simulink model "mainSimulink_localPi"  (R2021a)
settings: Solver=VariableStepAuto  StartTime=0.0  StopTime=inf  FixedStep=sensorSamplingTime  RelTol=1e-3
model workspace (MATLAB code in the model file):
  | %% Simulink settings
  | controllerFile = 'directFFcontroller';
  | set_param('mainSimulink_localPi/Subsystem Reference', 'ReferencedSubsystem', controllerFile);
  | %% Display settings
  | scopeTimeSpan = 30;
  | 
  | %% Robot settings (must match Python)
  | sensorFreq = 125;
  | actuatorFreq = 125;
  | TCPport = 12345;
  | dataSize = 4;
  | sensorSamplingTime = 1/sensorFreq;
  | actuatorTime = 1/actuatorFreq;
undefined symbols (not defined in the file): f
libraries: simulink x2, instrumentlib x2
settings Model: Creator=chukh  LastModifiedBy=brandon

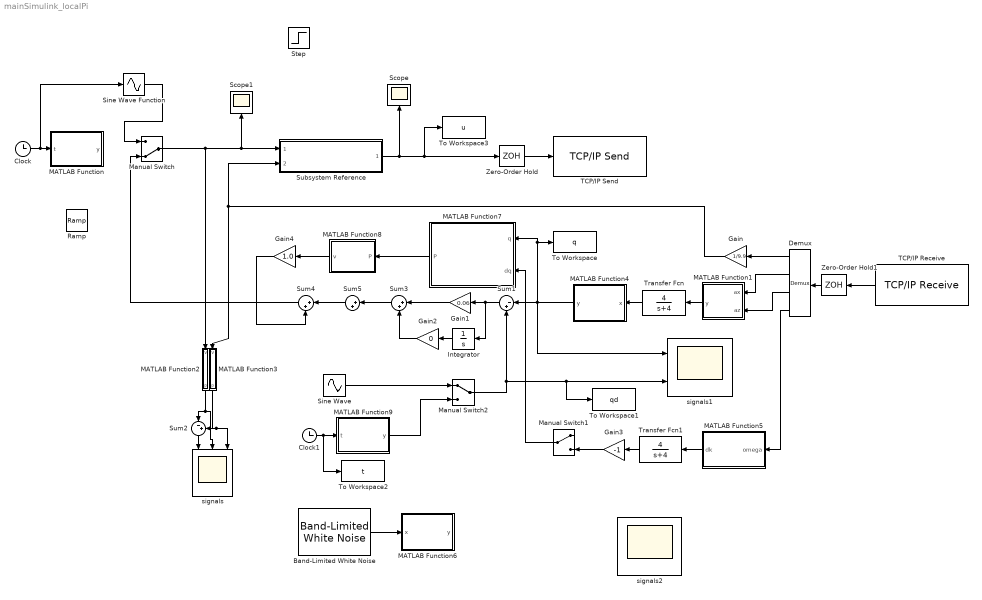
== system mainSimulink_localPi ==
  Band-Limited White Noise : simulink/Sources/Band-Limited White Noise  Cov=[0.1]  Ts=3  seed=[23341]
  Clock : Clock
  Clock1 : Clock
  Demux : Demux
  Gain : Gain  Gain=1/9.9
  Gain1 : Gain  Gain=0.06
  Gain2 : Gain  Gain=0
  Gain3 : Gain  Gain=-1
  Gain4 : Gain  Gain=1.0
  Integrator : Integrator
  MATLAB Function : MATLAB Function  TreatAsAtomicUnit=on
  MATLAB Function1 : MATLAB Function  TreatAsAtomicUnit=on
  MATLAB Function2 : MATLAB Function  TreatAsAtomicUnit=on
  MATLAB Function3 : MATLAB Function  TreatAsAtomicUnit=on
  MATLAB Function4 : MATLAB Function  TreatAsAtomicUnit=on
  MATLAB Function5 : MATLAB Function  TreatAsAtomicUnit=on
  MATLAB Function6 : MATLAB Function  TreatAsAtomicUnit=on
  MATLAB Function7 : MATLAB Function  TreatAsAtomicUnit=on
  MATLAB Function8 : MATLAB Function  TreatAsAtomicUnit=on
  MATLAB Function9 : MATLAB Function  TreatAsAtomicUnit=on
  Manual Switch : ManualSwitch  CurrentSetting=0
  Manual Switch1 : ManualSwitch
  Manual Switch2 : ManualSwitch
  Ramp : simulink/Sources/Ramp  slope=0.06  start=3  InitialOutput=0.6
  Scope : Scope
  Scope1 : Scope
  Sine Wave : Sin  Amplitude=8  Bias=8  Frequency=2  SampleTime=0
  Sine Wave Function : Sin  TimeSource=Use external signal  Amplitude=.4  Bias=0.5  Frequency=2  SampleTime=0
  Step : Step  Time=4  Before=0.6  After=0.85  SampleTime=0
  Subsystem Reference : Subsystem  ReferencedSubsystem=directFFcontroller
  Sum1 : Sum  Inputs=|-+
  Sum2 : Sum  Inputs=|-+
  Sum3 : Sum  Inputs=|++
  Sum4 : Sum  Inputs=|++
  Sum5 : Sum  Inputs=|++
  TCP/IP Receive : instrumentlib/TCP//IP Receive  Host=192.168.4.1  Port=12345  DataSize=dataSize  EnableBlockingMode=on  Timeout=0.5  SampleTime=sensorSamplingTime  DataType=double  ByteOrder=LittleEndian  ASCIIFormatting=%f,  Terminator=LF
  TCP/IP Send : instrumentlib/TCP//IP Send  Host=192.168.4.1  Port=12345  EnableBlockingMode=on  Timeout=0.5  ByteOrder=LittleEndian  TransferDelay=on
  To Workspace : ToWorkspace  VariableName=q  SaveFormat=Timeseries  SampleTime=-1
  To Workspace1 : ToWorkspace  VariableName=qd  SaveFormat=Timeseries  SampleTime=-1
  To Workspace2 : ToWorkspace  VariableName=t  SaveFormat=Timeseries  SampleTime=-1
  To Workspace3 : ToWorkspace  VariableName=u  SaveFormat=Timeseries  SampleTime=-1
  Transfer Fcn : TransferFcn  Numerator=[4]  Denominator=[1 4]
  Transfer Fcn1 : TransferFcn  Numerator=[4]  Denominator=[1 4]
  Zero-Order Hold : ZeroOrderHold  SampleTime=actuatorTime
  Zero-Order Hold1 : ZeroOrderHold  SampleTime=actuatorTime
  signals : Scope  NumInputPorts=3
  signals1 : Scope  NumInputPorts=2
  signals2 : Scope  NumInputPorts=2
  wires:
  Subsystem Reference/1 -> To Workspace3/1, Zero-Order Hold/1, Scope/1
  TCP/IP Receive/1 -> Zero-Order Hold1/1
  Zero-Order Hold/1 -> TCP/IP Send/1
  MATLAB Function2/1(p) -> Sum2/1, signals/2
  Gain/1 -> MATLAB Function3/1(V), Subsystem Reference/2
  MATLAB Function3/1(p) -> Sum2/2, signals/3
  Sum2/1 -> signals/1
  Clock/1 -> Sine Wave Function/1, MATLAB Function/1(t)
  Manual Switch/1 -> Scope1/1, Subsystem Reference/1, MATLAB Function2/1(V)
  Sine Wave Function/1 -> Manual Switch/1
  Demux/1 -> Gain/1
  Zero-Order Hold1/1 -> Demux/1
  Demux/2 -> MATLAB Function1/1(ax)
  MATLAB Function1/1(y) -> Transfer Fcn/1
  Transfer Fcn/1 -> MATLAB Function4/1(x)
  MATLAB Function4/1(y) -> MATLAB Function7/1(q), To Workspace/1, Sum1/1, signals1/1
  Sum1/1 -> Integrator/1, Gain1/1
  Integrator/1 -> Gain2/1
  Gain1/1 -> Sum3/1
  Gain2/1 -> Sum3/2
  Demux/3 -> MATLAB Function1/2(az)
  Sum4/1 -> Manual Switch/2
  Demux/4 -> MATLAB Function5/1(omega)
  MATLAB Function5/1(dk) -> Transfer Fcn1/1
  Band-Limited White Noise/1 -> MATLAB Function6/1(x)
  MATLAB Function7/1(P) -> MATLAB Function8/1(P)
  MATLAB Function8/1(v) -> Gain4/1
  Gain4/1 -> Sum4/2
  Sum3/1 -> Sum5/1
  Sum5/1 -> Sum4/1
  Manual Switch1/1 -> MATLAB Function7/2(dq)
  Gain3/1 -> Manual Switch1/2
  Transfer Fcn1/1 -> Gain3/1
  Sine Wave/1 -> Manual Switch2/1
  MATLAB Function9/1(y) -> Manual Switch2/2
  Manual Switch2/1 -> Sum1/2, To Workspace1/1, signals1/2
  Clock1/1 -> To Workspace2/1, MATLAB Function9/1(t)

== matlab function mainSimulink_localPi/MATLAB Function2 ==
  data: V input; p output
function p = V2kPa(V)
p = (V-0.5)*200;

== matlab function mainSimulink_localPi/MATLAB Function3 ==
  data: V input; p output
function p = V2kPa(V)
p = (V-0.5)*200;

== matlab function mainSimulink_localPi/MATLAB Function1 ==
  data: ax input; y output; az input
function y = fcn(ax,az)

y = -atan2(-az,-ax);

== matlab function mainSimulink_localPi/MATLAB Function4 ==
  data: x input; y output
function y = rad2kappa(x)
y = x/0.0875;
end

== matlab function mainSimulink_localPi/MATLAB Function5 ==
  data: omega input; dk output
function dk = fcn(omega)

dk = omega/0.085;

== matlab function mainSimulink_localPi/MATLAB Function6 ==
  data: x input; y output
function y = rad2kappa(x)
y = (0.5*x + 0.5)*10;
end

== matlab function mainSimulink_localPi/MATLAB Function7 ==
  data: q input; P output; dq input
function P = ModelBasedController(q,dq)
L = 0.085;
H = 1.060e-5;
K = NonlinearStiffness(q);
D = 2.5e-6;
m = 0.00015;

tau = K*L*q + D*dq + m*cos(L*q);
P   = tau/H;

end

% %% functions
% function tau = Controller(mdl,Y)
%  r1 = 1.060e-5;
%  ii = max(round((mdl.t)/mdl.Tstep),1);
%  tau =  r1*[0;0;Y(ii)];
% end

function k = NonlinearStiffness(x)
k = 5.62e-4*(exp((-min(x/12,0)))) + 3e-8*abs(min((x+2),0).*(x+2).^6);
end

== matlab function mainSimulink_localPi/MATLAB Function8 ==
  data: P input; v output
function v = kPa2V(P)
v = 0.5+(P/200);

== matlab function mainSimulink_localPi/MATLAB Function9 ==
  data: t input; y output
function y = fcn(t)

y = (6+5*sin(min(0.1*t,2)*t));

== matlab function mainSimulink_localPi/MATLAB Function ==
  data: t input; y output
function y = fcn(t)

y = (0.6+0.3*sin(0.25*t^2));
